simulink library "halout"  (R2021b)
settings: Solver=VariableStepAuto  StartTime=0.0  StopTime=10.0  RelTol=1e-3
undefined symbols (not defined in the file): C_TASK_5MS_S, FALSE, KHAL_CAN1FD1APS3E2E_flg, KHAL_CAN1FD1APS3TxReq_flg, KHAL_CAN1FD1VCU2E2E_flg, KHAL_CAN1FD1VCU2TxReq_flg, KHAL_CAN1FD1VCU3E2E_flg, KHAL_CAN1FD1VCU3TxReq_flg, KHAL_CAN1TxReq_flg, KHAL_CAN1VMCFCM1E2E_flg, KHAL_CAN1VMCFCM1TxReq_flg, KHAL_CAN2TxReq_flg, KHAL_CAN3FD3VCU1toNIDECTxReq_flg, KHAL_CAN3FD3VCU1TxReq_flg, KHAL_CAN3FD3VCU2E2E_flg, KHAL_CAN3FD3VCU2toNIDECE2E_flg, KHAL_CAN3FD3VCU2toNIDECTxReq_flg, KHAL_CAN3FD3VCU2TxReq_flg, KHAL_CAN3TxReq_flg, KHAL_CAN4FD4CE1000E2E_flg, KHAL_CAN4FD4CE1000TxReq_flg, KHAL_CAN4TxReq_flg, KHAL_CAN5TxReq_flg, KHAL_CAN6FD6APS3E2E_flg, KHAL_CAN6FD6APS3TxReq_flg, KHAL_CAN6FD6VCU2E2E_flg, KHAL_CAN6FD6VCU2TxReq_flg, KHAL_CAN6TxReq_flg, ONE_INT, TRUE, ZERO_INT
libraries: FVT_lib x551, simulink x244
(part 7 of 26)

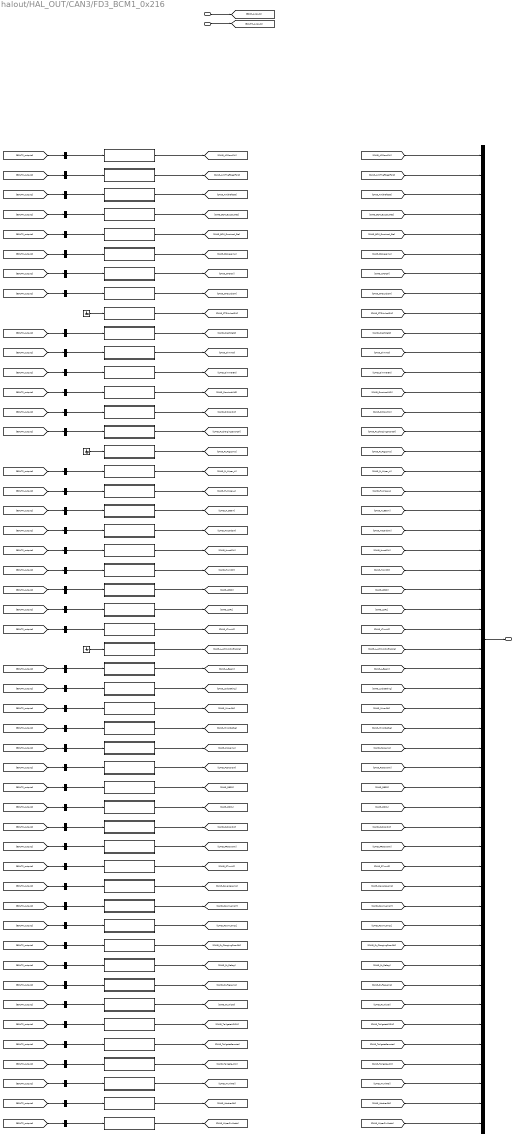
== system halout/HAL_OUT/CAN3/FD3_BCM1_0x216 ==
  BSCP_outputs : Inport  OutDataTypeStr=Bus: BSCP_outputs
  BOUTP_outputs : Inport  Port=2  OutDataTypeStr=Bus: BOUTP_outputs
  AllDoorSW : Subsystem
  AntiTheftSeatFold : Subsystem
  AntitheftSta : Subsystem
  BCMBuzzerReq : Subsystem
  BCMDoorLockSta : Subsystem
  BrakeLamp : Subsystem
  CTDCtrl : Subsystem
  CTDLockSW : Subsystem
  CTDUnlockSW : Subsystem
  CrashDetd : Subsystem
  Dimmer : Subsystem
  DimmerEN : Subsystem
  DoorLockIND : Subsystem
  DrDoorSW : Subsystem
  FrChargingDoorCtrl : Subsystem
  FrFogLamp : Subsystem
  FrWiperH : Subsystem
  FrWiperL : Subsystem
  Ground : Ground
  Ground1 : Ground
  Ground2 : Ground
  HBeam : Subsystem
  HazardSW : Subsystem
  HoodSW : Subsystem
  HornCtrl : Subsystem
  LAPMWdwEnable : Subsystem
  LBSD : Subsystem
  LBeam : Subsystem
  LDRL : Subsystem
  LTurnLP : Subsystem
  LockSetting : Subsystem
  MirrorCtrl : Subsystem
  MirrorDefog : Subsystem
  PosLamp : Subsystem
  PsDoorSW : Subsystem
  RBSD : Subsystem
  RDRL : Subsystem
  RLDoorSW : Subsystem
  RRDoorSW : Subsystem
  RTurnLP : Subsystem
  ReverseLamp : Subsystem
  RoomLampH : Subsystem
  RoomLampL : Subsystem
  RrChargingDoorCtrl : Subsystem
  RrDefog : Subsystem
  RrFogLamp : Subsystem
  RrWiper : Subsystem
  TailgateHDSW : Subsystem
  TailgateRemote : Subsystem
  TailgateSW : Subsystem
  TrunkRel : Subsystem
  WasherCtrl : Subsystem
  WiperFixMode : Subsystem
  bus_creator : BusCreator  Inputs=50  OutDataTypeStr=Bus: DT_CAN3_SG_FD3_BCM1  NonVirtualBus=on
  bus_selector : BusSelector  OutputSignals=VOUTP_AllDoorSW_flg
  bus_selector1 : BusSelector  OutputSignals=VOUTP_AntitheftSeatFlod_flg
  bus_selector10 : BusSelector  OutputSignals=VOUTP_DimmerEN_flg
  bus_selector11 : BusSelector  OutputSignals=VOUTP_DoorLockIND_flg
  bus_selector12 : BusSelector  OutputSignals=VOUTP_DrDoorSW_flg
  bus_selector13 : BusSelector  OutputSignals=VOUTP_FrChargingDoorCtrl_enum
  bus_selector14 : BusSelector  OutputSignals=VOUTP_FrWiperH_flg
  bus_selector15 : BusSelector  OutputSignals=VOUTP_FrWiperL_flg
  bus_selector16 : BusSelector  OutputSignals=VOUTP_HBeam_flg
  bus_selector17 : BusSelector  OutputSignals=VOUTP_HazardSW_flg
  bus_selector18 : BusSelector  OutputSignals=VOUTP_HoodSW_flg
  bus_selector19 : BusSelector  OutputSignals=VOUTP_HornCtrl_flg
  bus_selector2 : BusSelector  OutputSignals=VOUTP_AntitheftSta_enum
  bus_selector20 : BusSelector  OutputSignals=VOUTP_LBSD_flg
  bus_selector21 : BusSelector  OutputSignals=VOUTP_LDRL_flg
  bus_selector22 : BusSelector  OutputSignals=VOUTP_LTurnLP_flg
  bus_selector23 : BusSelector  OutputSignals=VOUTP_LBeam_flg
  bus_selector24 : BusSelector  OutputSignals=VOUTP_LockSetting_flg
  bus_selector25 : BusSelector  OutputSignals=VOUTP_MirrorCtrl_enum
  bus_selector26 : BusSelector  OutputSignals=VOUTP_MirrorDefog_flg
  bus_selector27 : BusSelector  OutputSignals=VOUTP_PosLamp_flg
  bus_selector28 : BusSelector  OutputSignals=VOUTP_PsDoorSW_flg
  bus_selector29 : BusSelector  OutputSignals=VOUTP_RBSD_flg
  bus_selector3 : BusSelector  OutputSignals=VOUTP_BCMBuzzerReq_flg
  bus_selector30 : BusSelector  OutputSignals=VOUTP_RDRL_flg
  bus_selector31 : BusSelector  OutputSignals=VOUTP_RLDoorSW_flg
  bus_selector32 : BusSelector  OutputSignals=VOUTP_RRDoorSW_flg
  bus_selector33 : BusSelector  OutputSignals=VOUTP_RTurnLP_flg
  bus_selector34 : BusSelector  OutputSignals=VOUTP_ReverseLamp_flg
  bus_selector35 : BusSelector  OutputSignals=VOUTP_RoomLampH_flg
  bus_selector36 : BusSelector  OutputSignals=VOUTP_RoomLampL_flg
  bus_selector37 : BusSelector  OutputSignals=VOUTP_RrChargingDoorCtrl_enum
  bus_selector38 : BusSelector  OutputSignals=VOUTP_RrDefog_flg
  bus_selector39 : BusSelector  OutputSignals=VOUTP_RrFogLamp_flg
  bus_selector4 : BusSelector  OutputSignals=VOUTP_BCMDoorLockSta_flg
  bus_selector40 : BusSelector  OutputSignals=VOUTP_RrWiper_flg
  bus_selector41 : BusSelector  OutputSignals=VOUTP_TailgateHDSW_flg
  bus_selector42 : BusSelector  OutputSignals=VOUTP_TailgateRemote_enum
  bus_selector43 : BusSelector  OutputSignals=VOUTP_TailgateSW_flg
  bus_selector44 : BusSelector  OutputSignals=VOUTP_TrunkRel_flg
  bus_selector45 : BusSelector  OutputSignals=VOUTP_WasherCtrl_enum
  bus_selector46 : BusSelector  OutputSignals=VOUTP_WiperFixMode_flg
  bus_selector5 : BusSelector  OutputSignals=VOUTP_BrakeLamp_flg
  bus_selector6 : BusSelector  OutputSignals=VOUTP_CTDCtrl_enum
  bus_selector7 : BusSelector  OutputSignals=VOUTP_CTDLockSW_flg
  bus_selector8 : BusSelector  OutputSignals=VOUTP_CrashDetd_flg
  bus_selector9 : BusSelector  OutputSignals=VOUTP_Dimmer_pct
  FD3_BCM1 : Outport
  wires:
  BSCP_outputs/1 -> [BSCP_outputs]
  BOUTP_outputs/1 -> [BOUTP_outputs]
  [CAN3_AllDoorSW] -> bus_creator/1  "CAN3_AllDoorSW"
  [CAN3_AntiTheftSeatFold] -> bus_creator/2  "CAN3_AntiTheftSeatFold"
  [CAN3_AntitheftSta] -> bus_creator/3  "CAN3_AntitheftSta"
  [CAN3_BCM_Buzzer_Req] -> bus_creator/4  "CAN3_BCM_Buzzer_Req"
  [CAN3_BCM_DoorLock_Sta] -> bus_creator/5  "CAN3_BCM_DoorLock_Sta"
  [CAN3_BrakeLamp] -> bus_creator/6  "CAN3_BrakeLamp"
  [CAN3_CTDCtrl] -> bus_creator/7  "CAN3_CTDCtrl"
  [CAN3_CTDLockSW] -> bus_creator/8  "CAN3_CTDLockSW"
  [CAN3_CTDUnlockSW] -> bus_creator/9  "CAN3_CTDUnlockSW"
  [CAN3_CrashDetd] -> bus_creator/10  "CAN3_CrashDetd"
  [CAN3_Dimmer] -> bus_creator/11  "CAN3_Dimmer"
  [CAN3_DimmerEN] -> bus_creator/12  "CAN3_DimmerEN"
  [CAN3_DoorLockIND] -> bus_creator/13  "CAN3_DoorLockIND"
  [CAN3_DrDoorSW] -> bus_creator/14  "CAN3_DrDoorSW"
  [CAN3_Fr_ChargingDoorCtrl] -> bus_creator/15  "CAN3_Fr_ChargingDoorCtrl"
  [CAN3_Fr_FogLamp] -> bus_creator/16  "CAN3_Fr_FogLamp"
  [CAN3_Fr_Wiper_H] -> bus_creator/17  "CAN3_Fr_Wiper_H"
  [CAN3_Fr_Wiper_L] -> bus_creator/18  "CAN3_Fr_Wiper_L"
  [CAN3_H_Beam] -> bus_creator/19  "CAN3_H_Beam"
  [CAN3_HazardSW] -> bus_creator/20  "CAN3_HazardSW"
  [CAN3_HoodSW] -> bus_creator/21  "CAN3_HoodSW"
  [CAN3_HornCtrl] -> bus_creator/22  "CAN3_HornCtrl"
  [CAN3_LBSD] -> bus_creator/23  "CAN3_LBSD"
  [CAN3_LDRL] -> bus_creator/24  "CAN3_LDRL"
  [CAN3_LTurnLP] -> bus_creator/25  "CAN3_LTurnLP"
  [CAN3_L_APM_WdwEnable] -> bus_creator/26  "CAN3_L_APM_WdwEnable"
  [CAN3_L_Beam] -> bus_creator/27  "CAN3_L_Beam"
  [CAN3_LockSetting] -> bus_creator/28  "CAN3_LockSetting"
  [CAN3_MirrorCtrl] -> bus_creator/29  "CAN3_MirrorCtrl"
  [CAN3_MirrorDefog] -> bus_creator/30  "CAN3_MirrorDefog"
  [CAN3_PosLamp] -> bus_creator/31  "CAN3_PosLamp"
  [CAN3_PsDoorSW] -> bus_creator/32  "CAN3_PsDoorSW"
  [CAN3_RBSD] -> bus_creator/33  "CAN3_RBSD"
  [CAN3_RDRL] -> bus_creator/34  "CAN3_RDRL"
  [CAN3_RLDoorSW] -> bus_creator/35  "CAN3_RLDoorSW"
  [CAN3_RRDoorSW] -> bus_creator/36  "CAN3_RRDoorSW"
  [CAN3_RTurnLP] -> bus_creator/37  "CAN3_RTurnLP"
  [CAN3_ReverseLamp] -> bus_creator/38  "CAN3_ReverseLamp"
  [CAN3_RoomLampH] -> bus_creator/39  "CAN3_RoomLampH"
  [CAN3_RoomLampL] -> bus_creator/40  "CAN3_RoomLampL"
  [CAN3_Rr_ChargingDoorCtrl] -> bus_creator/41  "CAN3_Rr_ChargingDoorCtrl"
  [CAN3_Rr_Defog] -> bus_creator/42  "CAN3_Rr_Defog"
  [CAN3_Rr_FogLamp] -> bus_creator/43  "CAN3_Rr_FogLamp"
  [CAN3_Rr_Wiper] -> bus_creator/44  "CAN3_Rr_Wiper"
  [CAN3_TailgateHDSW] -> bus_creator/45  "CAN3_TailgateHDSW"
  [CAN3_TailgateRemote] -> bus_creator/46  "CAN3_TailgateRemote"
  [CAN3_Tailgate_SW] -> bus_creator/47  "CAN3_Tailgate_SW"
  [CAN3_TrunkRel] -> bus_creator/48  "CAN3_TrunkRel"
  [CAN3_WasherCtrl] -> bus_creator/49  "CAN3_WasherCtrl"
  [CAN3_WiperFixMode] -> bus_creator/50  "CAN3_WiperFixMode"
  bus_creator/1 -> FD3_BCM1/1
  AllDoorSW/1(CAN3_AllDoorSW) -> [CAN3_AllDoorSW]
  AntiTheftSeatFold/1(CAN3_AntiTheftSeatFold) -> [CAN3_AntiTheftSeatFold]
  AntitheftSta/1(CAN3_AntitheftSta) -> [CAN3_AntitheftSta]
  BCMBuzzerReq/1(CAN3_BCM_Buzzer_Req) -> [CAN3_BCM_Buzzer_Req]
  BCMDoorLockSta/1(CAN3_BCM_DoorLock_Sta) -> [CAN3_BCM_DoorLock_Sta]
  BrakeLamp/1(CAN3_BrakeLamp) -> [CAN3_BrakeLamp]
  CTDCtrl/1(CAN3_CTDCtrl) -> [CAN3_CTDCtrl]
  CTDLockSW/1(CAN3_CTDLockSW) -> [CAN3_CTDLockSW]
  CTDUnlockSW/1(CAN3_CTDUnlockSW) -> [CAN3_CTDUnlockSW]
  CrashDetd/1(CAN3_CrashDetd) -> [CAN3_CrashDetd]
  Dimmer/1(CAN3_Dimmer) -> [CAN3_Dimmer]
  DimmerEN/1(CAN3_DimmerEN) -> [CAN3_DimmerEN]
  DoorLockIND/1(CAN3_DoorLockIND) -> [CAN3_DoorLockIND]
  DrDoorSW/1(CAN3_DrDoorSW) -> [CAN3_DrDoorSW]
  FrChargingDoorCtrl/1(CAN3_Fr_ChargingDoorCtrl) -> [CAN3_Fr_ChargingDoorCtrl]
  FrFogLamp/1(CAN3_Fr_FogLamp) -> [CAN3_Fr_FogLamp]
  FrWiperH/1(CAN3_Fr_Wiper_H) -> [CAN3_Fr_Wiper_H]
  FrWiperL/1(CAN3_Fr_Wiper_L) -> [CAN3_Fr_Wiper_L]
  HBeam/1(CAN3_H_Beam) -> [CAN3_H_Beam]
  HazardSW/1(CAN3_HazardSW) -> [CAN3_HazardSW]
  HoodSW/1(CAN3_HoodSW) -> [CAN3_HoodSW]
  HornCtrl/1(CAN3_HornCtrl) -> [CAN3_HornCtrl]
  LBSD/1(CAN3_LBSD) -> [CAN3_LBSD]
  LDRL/1(CAN3_LDRL) -> [CAN3_LDRL]
  LTurnLP/1(CAN3_LTurnLP) -> [CAN3_LTurnLP]
  LAPMWdwEnable/1(CAN3_L_APM_WdwEnable) -> [CAN3_L_APM_WdwEnable]
  LBeam/1(CAN3_L_Beam) -> [CAN3_L_Beam]
  LockSetting/1(CAN3_LockSetting) -> [CAN3_LockSetting]
  MirrorCtrl/1(CAN3_MirrorCtrl) -> [CAN3_MirrorCtrl]
  MirrorDefog/1(CAN3_MirrorDefog) -> [CAN3_MirrorDefog]
  PosLamp/1(CAN3_PosLamp) -> [CAN3_PosLamp]
  PsDoorSW/1(CAN3_PsDoorSW) -> [CAN3_PsDoorSW]
  RBSD/1(CAN3_RBSD) -> [CAN3_RBSD]
  RDRL/1(CAN3_RDRL) -> [CAN3_RDRL]
  RLDoorSW/1(CAN3_RLDoorSW) -> [CAN3_RLDoorSW]
  RRDoorSW/1(CAN3_RRDoorSW) -> [CAN3_RRDoorSW]
  RTurnLP/1(CAN3_RTurnLP) -> [CAN3_RTurnLP]
  ReverseLamp/1(CAN3_ReverseLamp) -> [CAN3_ReverseLamp]
  RoomLampH/1(CAN3_RoomLampH) -> [CAN3_RoomLampH]
  RoomLampL/1(CAN3_RoomLampL) -> [CAN3_RoomLampL]
  RrChargingDoorCtrl/1(CAN3_Rr_ChargingDoorCtrl) -> [CAN3_Rr_ChargingDoorCtrl]
  RrDefog/1(CAN3_Rr_Defog) -> [CAN3_Rr_Defog]
  RrFogLamp/1(CAN3_Rr_FogLamp) -> [CAN3_Rr_FogLamp]
  RrWiper/1(CAN3_Rr_Wiper) -> [CAN3_Rr_Wiper]
  TailgateHDSW/1(CAN3_TailgateHDSW) -> [CAN3_TailgateHDSW]
  TailgateRemote/1(CAN3_TailgateRemote) -> [CAN3_TailgateRemote]
  TailgateSW/1(CAN3_Tailgate_SW) -> [CAN3_Tailgate_SW]
  TrunkRel/1(CAN3_TrunkRel) -> [CAN3_TrunkRel]
  WasherCtrl/1(CAN3_WasherCtrl) -> [CAN3_WasherCtrl]
  WiperFixMode/1(CAN3_WiperFixMode) -> [CAN3_WiperFixMode]
  bus_selector/1 -> AllDoorSW/1(AllDoorSW)  "<VOUTP_AllDoorSW_flg>"
  [BOUTP_outputs] -> bus_selector/1
  bus_selector1/1 -> AntiTheftSeatFold/1(AntiTheftSeatFold)  "<VOUTP_AntitheftSeatFlod_flg>"
  [BOUTP_outputs] -> bus_selector1/1
  bus_selector2/1 -> AntitheftSta/1(AntitheftSta)  "<VOUTP_AntitheftSta_enum>"
  [BOUTP_outputs] -> bus_selector2/1
  bus_selector3/1 -> BCMBuzzerReq/1(BCMBuzzerReq)  "<VOUTP_BCMBuzzerReq_flg>"
  [BOUTP_outputs] -> bus_selector3/1
  bus_selector4/1 -> BCMDoorLockSta/1(BCMDoorLockSta)  "<VOUTP_BCMDoorLockSta_flg>"
  [BOUTP_outputs] -> bus_selector4/1
  bus_selector5/1 -> BrakeLamp/1(BrakeLamp)  "<VOUTP_BrakeLamp_flg>"
  [BOUTP_outputs] -> bus_selector5/1
  bus_selector6/1 -> CTDCtrl/1(CTDCtrl)  "<VOUTP_CTDCtrl_enum>"
  [BOUTP_outputs] -> bus_selector6/1
  bus_selector7/1 -> CTDLockSW/1(CTDLockSW)  "<VOUTP_CTDLockSW_flg>"
  [BOUTP_outputs] -> bus_selector7/1
  Ground/1 -> CTDUnlockSW/1(CTDUnlockSW)
  bus_selector8/1 -> CrashDetd/1(CrashDetd)  "<VOUTP_CrashDetd_flg>"
  [BOUTP_outputs] -> bus_selector8/1
  bus_selector9/1 -> Dimmer/1(Dimmer)  "<VOUTP_Dimmer_pct>"
  [BOUTP_outputs] -> bus_selector9/1
  bus_selector10/1 -> DimmerEN/1(DimmerEN)  "<VOUTP_DimmerEN_flg>"
  [BOUTP_outputs] -> bus_selector10/1
  bus_selector11/1 -> DoorLockIND/1(DoorLockIND)  "<VOUTP_DoorLockIND_flg>"
  [BOUTP_outputs] -> bus_selector11/1
  bus_selector12/1 -> DrDoorSW/1(DrDoorSW)  "<VOUTP_DrDoorSW_flg>"
  [BOUTP_outputs] -> bus_selector12/1
  bus_selector13/1 -> FrChargingDoorCtrl/1(FrChargingDoorCtrl)  "<VOUTP_FrChargingDoorCtrl_enum>"
  [BOUTP_outputs] -> bus_selector13/1
  Ground1/1 -> FrFogLamp/1(FrFogLamp)
  bus_selector14/1 -> FrWiperH/1(FrWiperH)  "<VOUTP_FrWiperH_flg>"
  [BOUTP_outputs] -> bus_selector14/1
  bus_selector15/1 -> FrWiperL/1(FrWiperL)  "<VOUTP_FrWiperL_flg>"
  [BOUTP_outputs] -> bus_selector15/1
  bus_selector16/1 -> HBeam/1(HBeam)  "<VOUTP_HBeam_flg>"
  [BOUTP_outputs] -> bus_selector16/1
  bus_selector17/1 -> HazardSW/1(HazardSW)  "<VOUTP_HazardSW_flg>"
  [BOUTP_outputs] -> bus_selector17/1
  bus_selector18/1 -> HoodSW/1(HoodSW)  "<VOUTP_HoodSW_flg>"
  [BOUTP_outputs] -> bus_selector18/1
  bus_selector19/1 -> HornCtrl/1(HornCtrl)  "<VOUTP_HornCtrl_flg>"
  [BOUTP_outputs] -> bus_selector19/1
  bus_selector20/1 -> LBSD/1(LBSD)  "<VOUTP_LBSD_flg>"
  [BOUTP_outputs] -> bus_selector20/1
  bus_selector21/1 -> LDRL/1(LDRL)  "<VOUTP_LDRL_flg>"
  [BOUTP_outputs] -> bus_selector21/1
  bus_selector22/1 -> LTurnLP/1(LTurnLP)  "<VOUTP_LTurnLP_flg>"
  [BOUTP_outputs] -> bus_selector22/1
  Ground2/1 -> LAPMWdwEnable/1(LAPMWdwEnable)
  bus_selector23/1 -> LBeam/1(LBeam)  "<VOUTP_LBeam_flg>"
  [BOUTP_outputs] -> bus_selector23/1
  bus_selector24/1 -> LockSetting/1(LockSetting)  "<VOUTP_LockSetting_flg>"
  [BOUTP_outputs] -> bus_selector24/1
  bus_selector25/1 -> MirrorCtrl/1(MirrorCtrl)  "<VOUTP_MirrorCtrl_enum>"
  [BOUTP_outputs] -> bus_selector25/1
  bus_selector26/1 -> MirrorDefog/1(MirrorDefog)  "<VOUTP_MirrorDefog_flg>"
  [BOUTP_outputs] -> bus_selector26/1
  bus_selector27/1 -> PosLamp/1(PosLamp)  "<VOUTP_PosLamp_flg>"
  [BOUTP_outputs] -> bus_selector27/1
  bus_selector28/1 -> PsDoorSW/1(PsDoorSW)  "<VOUTP_PsDoorSW_flg>"
  [BOUTP_outputs] -> bus_selector28/1
  bus_selector29/1 -> RBSD/1(RBSD)  "<VOUTP_RBSD_flg>"
  [BOUTP_outputs] -> bus_selector29/1
  bus_selector30/1 -> RDRL/1(RDRL)  "<VOUTP_RDRL_flg>"
  [BOUTP_outputs] -> bus_selector30/1
  bus_selector31/1 -> RLDoorSW/1(RLDoorSW)  "<VOUTP_RLDoorSW_flg>"
  [BOUTP_outputs] -> bus_selector31/1
  bus_selector32/1 -> RRDoorSW/1(RRDoorSW)  "<VOUTP_RRDoorSW_flg>"
  [BOUTP_outputs] -> bus_selector32/1
  bus_selector33/1 -> RTurnLP/1(RTurnLP)  "<VOUTP_RTurnLP_flg>"
  [BOUTP_outputs] -> bus_selector33/1
  bus_selector34/1 -> ReverseLamp/1(ReverseLamp)  "<VOUTP_ReverseLamp_flg>"
  [BOUTP_outputs] -> bus_selector34/1
  bus_selector35/1 -> RoomLampH/1(RoomLampH)  "<VOUTP_RoomLampH_flg>"
  [BOUTP_outputs] -> bus_selector35/1
  bus_selector36/1 -> RoomLampL/1(RoomLampL)  "<VOUTP_RoomLampL_flg>"
  [BOUTP_outputs] -> bus_selector36/1
  bus_selector37/1 -> RrChargingDoorCtrl/1(RrChargingDoorCtrl)  "<VOUTP_RrChargingDoorCtrl_enum>"
  [BOUTP_outputs] -> bus_selector37/1
  bus_selector38/1 -> RrDefog/1(RrDefog)  "<VOUTP_RrDefog_flg>"
  [BOUTP_outputs] -> bus_selector38/1
  bus_selector39/1 -> RrFogLamp/1(RrFogLamp)  "<VOUTP_RrFogLamp_flg>"
  [BOUTP_outputs] -> bus_selector39/1
  bus_selector40/1 -> RrWiper/1(RrWiper)  "<VOUTP_RrWiper_flg>"
  [BOUTP_outputs] -> bus_selector40/1
  bus_selector41/1 -> TailgateHDSW/1(TailgateHDSW)  "<VOUTP_TailgateHDSW_flg>"
  [BOUTP_outputs] -> bus_selector41/1
  bus_selector42/1 -> TailgateRemote/1(TailgateRemote)  "<VOUTP_TailgateRemote_enum>"
  [BOUTP_outputs] -> bus_selector42/1
  bus_selector43/1 -> TailgateSW/1(TailgateSW)  "<VOUTP_TailgateSW_flg>"
  [BOUTP_outputs] -> bus_selector43/1
  bus_selector44/1 -> TrunkRel/1(TrunkRel)  "<VOUTP_TrunkRel_flg>"
  [BOUTP_outputs] -> bus_selector44/1
  bus_selector45/1 -> WasherCtrl/1(WasherCtrl)  "<VOUTP_WasherCtrl_enum>"
  [BOUTP_outputs] -> bus_selector45/1
  bus_selector46/1 -> WiperFixMode/1(WiperFixMode)  "<VOUTP_WiperFixMode_flg>"
  [BOUTP_outputs] -> bus_selector46/1

== system halout/HAL_OUT/CAN3/FD3_C100_0_0x182 ==
  BSCP_outputs : Inport  OutDataTypeStr=Bus: BSCP_outputs
  BOUTP_outputs : Inport  Port=2  OutDataTypeStr=Bus: BOUTP_outputs
  BatteryMode : Subsystem
  FrCoolantflow : Subsystem
  FrCoolanttemp : Subsystem
  Ground{,1..4} (5 alike) : Ground
  RrCoolantflow : Subsystem
  RrCoolanttemp : Subsystem
  bus_creator : BusCreator  Inputs=6  OutDataTypeStr=Bus: DT_CAN3_SG_FD3_C100_0  NonVirtualBus=on
  bus_selector : BusSelector  OutputSignals=VOUTP_BatteryMode_enum
  sigCbnPTCPwrAct : Subsystem
  FD3_C100_0 : Outport
  wires:
  BSCP_outputs/1 -> [BSCP_outputs]
  BOUTP_outputs/1 -> [BOUTP_outputs]
  [CAN3_BatteryMode] -> bus_creator/1  "CAN3_BatteryMode"
  [CAN3_Fr_Coolantflow] -> bus_creator/2  "CAN3_Fr_Coolantflow"
  [CAN3_Fr_Coolanttemp] -> bus_creator/3  "CAN3_Fr_Coolanttemp"
  [CAN3_Rr_Coolantflow] -> bus_creator/4  "CAN3_Rr_Coolantflow"
  [CAN3_Rr_Coolanttemp] -> bus_creator/5  "CAN3_Rr_Coolanttemp"
  [CAN3_sigCbnPTCPwrAct] -> bus_creator/6  "CAN3_sigCbnPTCPwrAct"
  bus_creator/1 -> FD3_C100_0/1
  BatteryMode/1(CAN3_BatteryMode) -> [CAN3_BatteryMode]
  FrCoolantflow/1(CAN3_Fr_Coolantflow) -> [CAN3_Fr_Coolantflow]
  FrCoolanttemp/1(CAN3_Fr_Coolanttemp) -> [CAN3_Fr_Coolanttemp]
  RrCoolantflow/1(CAN3_Rr_Coolantflow) -> [CAN3_Rr_Coolantflow]
  RrCoolanttemp/1(CAN3_Rr_Coolanttemp) -> [CAN3_Rr_Coolanttemp]
  sigCbnPTCPwrAct/1(CAN3_sigCbnPTCPwrAct) -> [CAN3_sigCbnPTCPwrAct]
  bus_selector/1 -> BatteryMode/1(BatteryMode)  "<VOUTP_BatteryMode_enum>"
  [BOUTP_outputs] -> bus_selector/1
  Ground/1 -> FrCoolantflow/1(FrCoolantflow)
  Ground1/1 -> FrCoolanttemp/1(FrCoolanttemp)
  Ground2/1 -> RrCoolantflow/1(RrCoolantflow)
  Ground3/1 -> RrCoolanttemp/1(RrCoolanttemp)
  Ground4/1 -> sigCbnPTCPwrAct/1(sigCbnPTCPwrAct)

== system halout/HAL_OUT/CAN3/FD3_V2L1_0x374 ==
  BSCP_outputs : Inport  OutDataTypeStr=Bus: BSCP_outputs
  BOUTP_outputs : Inport  Port=2  OutDataTypeStr=Bus: BOUTP_outputs
  FDCV2LOBCExtrV2LCmd : Subsystem
  FDCV2LOBCIntrV2LCmd : Subsystem
  Ground : Ground
  ReqOBCV2LEna : Subsystem
  ReqV2LIVIPopup : Subsystem
  ReqV2LSwOn : Subsystem
  bus_creator : BusCreator  Inputs=5  OutDataTypeStr=Bus: DT_CAN3_SG_FD3_V2L1  NonVirtualBus=on
  bus_selector : BusSelector  OutputSignals=VOUTP_ReqOBCExtrV2LEna_enum
  bus_selector1 : BusSelector  OutputSignals=VOUTP_ReqOBCIntrV2LEna_enum
  bus_selector2 : BusSelector  OutputSignals=VOUTP_ReqOBCV2LEna_enum
  bus_selector3 : BusSelector  OutputSignals=VOUTP_ReqV2LIVIPopup_enum
  FD3_V2L1 : Outport
  wires:
  BSCP_outputs/1 -> [BSCP_outputs]
  BOUTP_outputs/1 -> [BOUTP_outputs]
  [CAN3_FDC_V2L_OBCExtrV2L_Cmd] -> bus_creator/1  "CAN3_FDC_V2L_OBCExtrV2L_Cmd"
  [CAN3_FDC_V2L_OBCIntrV2L_Cmd] -> bus_creator/2  "CAN3_FDC_V2L_OBCIntrV2L_Cmd"
  [CAN3_Req_OBCV2LEna] -> bus_creator/3  "CAN3_Req_OBCV2LEna"
  [CAN3_Req_V2LSwOn] -> bus_creator/4  "CAN3_Req_V2LSwOn"
  [CAN3_Req_V2L_IVI_Popup] -> bus_creator/5  "CAN3_Req_V2L_IVI_Popup"
  bus_creator/1 -> FD3_V2L1/1
  FDCV2LOBCExtrV2LCmd/1(CAN3_FDC_V2L_OBCExtrV2L_Cmd) -> [CAN3_FDC_V2L_OBCExtrV2L_Cmd]
  FDCV2LOBCIntrV2LCmd/1(CAN3_FDC_V2L_OBCIntrV2L_Cmd) -> [CAN3_FDC_V2L_OBCIntrV2L_Cmd]
  ReqOBCV2LEna/1(CAN3_Req_OBCV2LEna) -> [CAN3_Req_OBCV2LEna]
  ReqV2LSwOn/1(CAN3_Req_V2LSwOn) -> [CAN3_Req_V2LSwOn]
  ReqV2LIVIPopup/1(CAN3_Req_V2L_IVI_Popup) -> [CAN3_Req_V2L_IVI_Popup]
  bus_selector/1 -> FDCV2LOBCExtrV2LCmd/1(FDCV2LOBCExtrV2LCmd)  "<VOUTP_ReqOBCExtrV2LEna_enum>"
  [BOUTP_outputs] -> bus_selector/1
  bus_selector1/1 -> FDCV2LOBCIntrV2LCmd/1(FDCV2LOBCIntrV2LCmd)  "<VOUTP_ReqOBCIntrV2LEna_enum>"
  [BOUTP_outputs] -> bus_selector1/1
  bus_selector2/1 -> ReqOBCV2LEna/1(ReqOBCV2LEna)  "<VOUTP_ReqOBCV2LEna_enum>"
  [BOUTP_outputs] -> bus_selector2/1
  Ground/1 -> ReqV2LSwOn/1(ReqV2LSwOn)
  bus_selector3/1 -> ReqV2LIVIPopup/1(ReqV2LIVIPopup)  "<VOUTP_ReqV2LIVIPopup_enum>"
  [BOUTP_outputs] -> bus_selector3/1

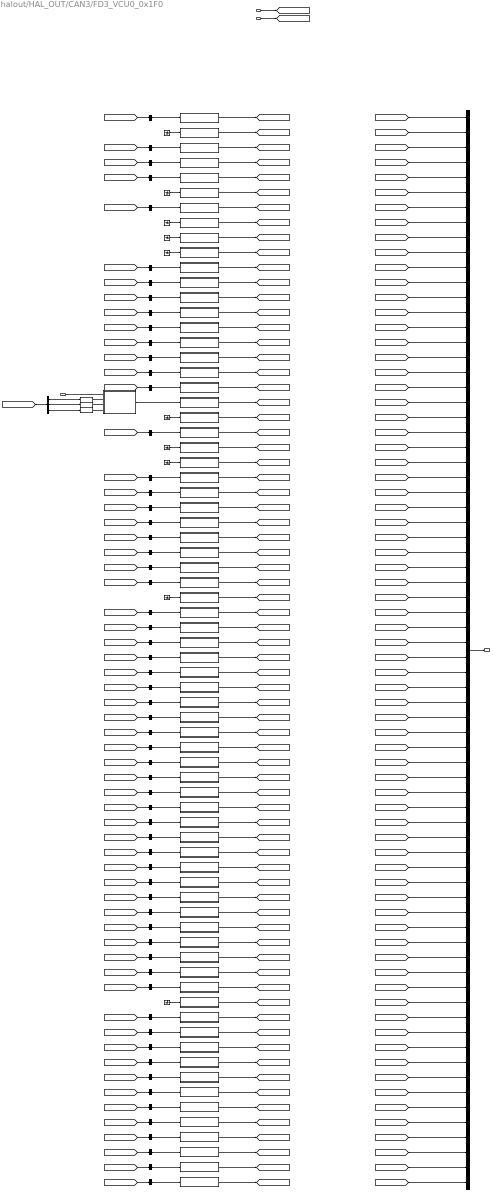
== system halout/HAL_OUT/CAN3/FD3_VCU0_0x1F0 ==
  BSCP_outputs : Inport  OutDataTypeStr=Bus: BSCP_outputs
  BOUTP_outputs : Inport  Port=2  OutDataTypeStr=Bus: BOUTP_outputs
  s8_AcoreReadyToSleep : Inport  Port=3
  Data Type Conversion : DataTypeConversion  OutDataTypeStr=uint8
  Data Type Conversion1 : DataTypeConversion  OutDataTypeStr=uint8
  Data Type Conversion2 : DataTypeConversion  OutDataTypeStr=uint8
  EVCCAplusPwrUpReq : Subsystem
  FDADC12VDet : Subsystem
  FDADC12VDetAvg : Subsystem
  FDCSYSPmicBootPath : Subsystem
  FDCVCUActMaxSlideRateSta : Subsystem
  FDCVCUAllowMovThdOTASta : Subsystem
  FDCVCUBOSEnableSta : Subsystem
  FDCVCUBrakeSigMatrixSta : Subsystem
  FDCVCUBrkPedalPosStaSta : Subsystem
  FDCVCUCANBrkSW2StaSta : Subsystem
  FDCVCUDTCCarouselSta : Subsystem
  FDCVCUEAPS1MinSta : Subsystem
  FDCVCUEAPS1RawSta : Subsystem
  FDCVCUEAPS2MinSta : Subsystem
  FDCVCUEAPS2RawSta : Subsystem
  FDCVCUForcePCmd : Subsystem
  FDCVCUFrFirstOrderInpTs : Subsystem
  FDCVCUFrRateLimitDecSta : Subsystem
  FDCVCUFrRateLimitIncSta : Subsystem
  FDCVCULVChrgFreqCntSta : Subsystem
  FDCVCULVStaDropQukCntSta : Subsystem
  FDCVCULowIdleAccPedalSta : Subsystem
  FDCVCUOTAPwrReqOFFChkSta : Subsystem
  FDCVCUOTAPwrReqStdChkSta : Subsystem
  FDCVCUPwrReqOTASta : Subsystem
  FDCVCURWDRDCActiveSta : Subsystem
  FDCVCURegenTqLimitEnSta : Subsystem
  FDCVCURrFirstOrderInpTs : Subsystem
  FDCVCURrRateLimitDecSta : Subsystem
  FDCVCURrRateLimitIncSta : Subsystem
  FDCVCUSlideRegenLimTqSta : Subsystem
  FDCVCUVehActSpdSta : Subsystem
  FDCVCUVehMalfunLevelSta : Subsystem
  FDCVMCActStESCYawSta : Subsystem
  FDCVMCLongAccSta : Subsystem
  FrTqSource : Subsystem
  Ground{,1..4,8..12} (10 alike) : Ground
  HVRlyOpFail : Subsystem
  HVTHCMSysAvail : Subsystem
  LVBattChrgtimeAct : Subsystem
  LVBattVoltSta : Subsystem
  LVChrgHoldTAct : Subsystem
  LVSilentChrgLv : Subsystem
  LVSilentChrgReq : Subsystem
  LVSilentChrgSta : Subsystem
  MCUActDisFail : Subsystem
  PMMAllowECUSleep : Subsystem
  PmicBootReason : Subsystem
  PowerDownFault : Subsystem
  PowerDownState : Subsystem
  PowerUpFault : Subsystem
  PowerUpState : Subsystem
  PwrDownReq : Subsystem
  PwrStaConstraint : Subsystem
  PwrStaONTOIVIPopReq : Subsystem
  PwrStaONTOIVIPopT : Subsystem
  PwrStaSelect : Subsystem
  PwrStaTOSta : Subsystem
  PwrUpReq : Subsystem
  RrTqSource : Subsystem
  SchedChgTOSta : Subsystem
  SilentChkAllowSleep : Subsystem
  Subsystem : Subsystem
  SysAllowReadySta : Subsystem
  SysPwrSta : Subsystem
  TCountSta : Subsystem
  TimerAllowSleep : Subsystem
  VCUBrkSWSta : Subsystem
  VCUFLDoorSta : Subsystem
  VCUFRDoorSta : Subsystem
  VCURLDoorSta : Subsystem
  VCURRDoorSta : Subsystem
  VehHVPwrAvail4THCM : Subsystem
  WisrBootReason : Subsystem
  bus_creator : BusCreator  Inputs=72  OutDataTypeStr=Bus: DT_CAN3_SG_FD3_VCU0  NonVirtualBus=on
  bus_selector : BusSelector  OutputSignals=VOUTP_EvccAplusPwrUpReq_flg
  bus_selector1 : BusSelector  OutputSignals=VOUTP_FDADC12VDetAvg_mV
  bus_selector10 : BusSelector  OutputSignals=VOUTP_FrRateLimitDec_Nm
  bus_selector11 : BusSelector  OutputSignals=VOUTP_FrRateLimitInc_Nm
  bus_selector12 : BusSelector  OutputSignals=VOUTP_LowIdleAccPedal_flg
  bus_selector13 : BusSelector  OutputSignals=VOUTP_PwrReq_OTA_enum
  bus_selector14 : BusSelector  OutputSignals=VOUTP_RDCActive_enum
  bus_selector15 : BusSelector  OutputSignals=VOUTP_RegenTqLimitEn_flg
  bus_selector16 : BusSelector  OutputSignals=VOUTP_RrFirstOrderInpTs_c
  bus_selector17 : BusSelector  OutputSignals=VOUTP_RrRateLimitDec_Nm
  bus_selector18 : BusSelector  OutputSignals=VOUTP_RrRateLimitInc_Nm
  bus_selector19 : BusSelector  OutputSignals=VOUTP_SlideRegenLimTq_Nm
  bus_selector2 : BusSelector  OutputSignals=VOUTP_PmicBootPath_raw32
  bus_selector20 : BusSelector  OutputSignals=VOUTP_VehActSpd_kph
  bus_selector21 : BusSelector  OutputSignals=VOUTP_ActStESCYaw_Dps
  bus_selector22 : BusSelector  OutputSignals=VOUTP_LongAcc_Gps
  bus_selector23 : BusSelector  OutputSignals=VOUTP_TqSourceFr_enum
  bus_selector24 : BusSelector  OutputSignals=VOUTP_HVRlyOpFail_flg
  bus_selector25 : BusSelector  OutputSignals=VOUTP_HVTHCMSysAvail_enum
  bus_selector26 : BusSelector  OutputSignals=VOUTP_LVBattChrgTimeCnt_s
  bus_selector27 : BusSelector  OutputSignals=VOUTP_LVBattVoltSta_enum
  bus_selector28 : BusSelector  OutputSignals=VOUTP_LVChrgHoldTtimer_s
  bus_selector29 : BusSelector  OutputSignals=VOUTP_LVSilentChrgLv_enum
  bus_selector3 : BusSelector  OutputSignals=VOUTP_MaxWhlSlideRate_pct
  bus_selector30 : BusSelector  OutputSignals=VOUTP_LVSilentChrgReq_flg
  bus_selector31 : BusSelector  OutputSignals=VOUTP_LVSilentChrgSta_enum
  bus_selector32 : BusSelector  OutputSignals=VOUTP_MCUActDisFail_flg
  bus_selector33 : BusSelector  OutputSignals=VOUTP_PMMAllowECUSleep_flg
  bus_selector34 : BusSelector  OutputSignals=VOUTP_PmicBootReason_enum
  bus_selector35 : BusSelector  OutputSignals=VOUTP_PowerDownFault_enum
  bus_selector36 : BusSelector  OutputSignals=VOUTP_PowerDownState_enum
  bus_selector37 : BusSelector  OutputSignals=VOUTP_PowerUpFault_enum
  bus_selector38 : BusSelector  OutputSignals=VOUTP_PowerUpState_enum
  bus_selector39 : BusSelector  OutputSignals=VOUTP_PwrDownReq_enum
  bus_selector4 : BusSelector  OutputSignals=VOUTP_BOSEnable_flg
  bus_selector40 : BusSelector  OutputSignals=VOUTP_PwrStaConstraint_enum
  bus_selector41 : BusSelector  OutputSignals=VOUTP_PwrStaONTOPopReq_flg
  bus_selector42 : BusSelector  OutputSignals=VOUTP_IVIPwrStaONTOPopT_s
  bus_selector43 : BusSelector  OutputSignals=VOUTP_PwrStaSelect_enum
  bus_selector44 : BusSelector  OutputSignals=VOUTP_PwrStaTOSta_enum
  bus_selector45 : BusSelector  OutputSignals=VOUTP_PwrUpReq_enum
  bus_selector46 : BusSelector  OutputSignals=VOUTP_TqSourceRr_enum
  bus_selector47 : BusSelector  OutputSignals=VOUTP_SilentChkAllowSleep_flg
  bus_selector48 : BusSelector  OutputSignals=VOUTP_SysAllowReadySta_flg
  bus_selector49 : BusSelector  OutputSignals=VOUTP_SysPowerMode_enum
  bus_selector5 : BusSelector  OutputSignals=VOUTP_DTCDetect_enum
  bus_selector50 : BusSelector  OutputSignals=VOUTP_TCountSta_enum
  bus_selector51 : BusSelector  OutputSignals=VOUTP_TimerAllowSleep_flg
  bus_selector52 : BusSelector  OutputSignals=VOUTP_VCUBrkSWSta_enum
  bus_selector53 : BusSelector  OutputSignals=VOUTP_VCUFLDoorSta_flg
  bus_selector54 : BusSelector  OutputSignals=VOUTP_VCUFRDoorSta_flg
  bus_selector55 : BusSelector  OutputSignals=VOUTP_VCURLDoorSta_flg
  bus_selector56 : BusSelector  OutputSignals=VOUTP_VCURRDoorSta_flg
  bus_selector57 : BusSelector  OutputSignals=VOUTP_VehHVPwrAvail4THCM_W
  bus_selector58 : BusSelector  OutputSignals=VOUTP_WisrBootReason_raw32
  bus_selector59 : BusSelector  OutputSignals=VOUTP_CurrentNmState_enum,VOUTP_OTAPwrReqOFFChkSta_enum,VOUTP_OTAPwrReqStdChkSta_enum
  bus_selector6 : BusSelector  OutputSignals=VOUTP_EAPS1MIN_pct
  bus_selector60 : BusSelector  OutputSignals=VOUTP_EAPS2RAW_pct
  bus_selector61 : BusSelector  OutputSignals=VOUTP_EAPS1RAW_pct
  bus_selector7 : BusSelector  OutputSignals=VOUTP_EAPS2MIN_pct
  bus_selector8 : BusSelector  OutputSignals=VOUTP_ForceP_flg
  bus_selector9 : BusSelector  OutputSignals=VOUTP_FrFirstOrderInpTs_c
  FD3_VCU0 : Outport
  wires:
  BSCP_outputs/1 -> [BSCP_outputs]
  BOUTP_outputs/1 -> [BOUTP_outputs]
  [CAN3_EVCCAplusPwrUpReq] -> bus_creator/1  "CAN3_EVCCAplusPwrUpReq"
  [CAN3_FDADC12VDet] -> bus_creator/2  "CAN3_FDADC12VDet"
  [CAN3_FDADC12VDetAvg] -> bus_creator/3  "CAN3_FDADC12VDetAvg"
  [CAN3_FDC_SYS_PmicBootPath] -> bus_creator/4  "CAN3_FDC_SYS_PmicBootPath"
  [CAN3_FDC_VCU_ActMaxSlideRate_Sta] -> bus_creator/5  "CAN3_FDC_VCU_ActMaxSlideRate_Sta"
  [CAN3_FDC_VCU_AllowMovThd_OTA_Sta] -> bus_creator/6  "CAN3_FDC_VCU_AllowMovThd_OTA_Sta"
  [CAN3_FDC_VCU_BOSEnable_Sta] -> bus_creator/7  "CAN3_FDC_VCU_BOSEnable_Sta"
  [CAN3_FDC_VCU_BrakeSigMatrix_Sta] -> bus_creator/8  "CAN3_FDC_VCU_BrakeSigMatrix_Sta"
  [CAN3_FDC_VCU_BrkPedalPosSta_Sta] -> bus_creator/9  "CAN3_FDC_VCU_BrkPedalPosSta_Sta"
  [CAN3_FDC_VCU_CANBrkSW2Sta_Sta] -> bus_creator/10  "CAN3_FDC_VCU_CANBrkSW2Sta_Sta"
  [CAN3_FDC_VCU_DTCCarousel_Sta] -> bus_creator/11  "CAN3_FDC_VCU_DTCCarousel_Sta"
  [CAN3_FDC_VCU_EAPS1Min_Sta] -> bus_creator/12  "CAN3_FDC_VCU_EAPS1Min_Sta"
  [CAN3_FDC_VCU_EAPS1Raw_Sta] -> bus_creator/13  "CAN3_FDC_VCU_EAPS1Raw_Sta"
  [CAN3_FDC_VCU_EAPS2Min_Sta] -> bus_creator/14  "CAN3_FDC_VCU_EAPS2Min_Sta"
  [CAN3_FDC_VCU_EAPS2Raw_Sta] -> bus_creator/15  "CAN3_FDC_VCU_EAPS2Raw_Sta"
  [CAN3_FDC_VCU_ForceP_Cmd] -> bus_creator/16  "CAN3_FDC_VCU_ForceP_Cmd"
  [CAN3_FDC_VCU_FrFirstOrderInpTs] -> bus_creator/17  "CAN3_FDC_VCU_FrFirstOrderInpTs"
  [CAN3_FDC_VCU_FrRateLimitDec_Sta] -> bus_creator/18  "CAN3_FDC_VCU_FrRateLimitDec_Sta"
  [CAN3_FDC_VCU_FrRateLimitInc_Sta] -> bus_creator/19  "CAN3_FDC_VCU_FrRateLimitInc_Sta"
  [CAN3_FDC_VCU_LVChrgFreqCnt_Sta] -> bus_creator/20  "CAN3_FDC_VCU_LVChrgFreqCnt_Sta"
  [CAN3_FDC_VCU_LVStaDropQukCnt_Sta] -> bus_creator/21  "CAN3_FDC_VCU_LVStaDropQukCnt_Sta"
  [CAN3_FDC_VCU_LowIdleAccPedal_Sta] -> bus_creator/22  "CAN3_FDC_VCU_LowIdleAccPedal_Sta"
  [CAN3_FDC_VCU_OTAPwrReqOFFChk_Sta] -> bus_creator/23  "CAN3_FDC_VCU_OTAPwrReqOFFChk_Sta"
  [CAN3_FDC_VCU_OTAPwrReqStdChk_Sta] -> bus_creator/24  "CAN3_FDC_VCU_OTAPwrReqStdChk_Sta"
  [CAN3_FDC_VCU_PwrReq_OTA_Sta] -> bus_creator/25  "CAN3_FDC_VCU_PwrReq_OTA_Sta"
  [CAN3_FDC_VCU_RWDRDCActive_Sta] -> bus_creator/26  "CAN3_FDC_VCU_RWDRDCActive_Sta"
  [CAN3_FDC_VCU_RegenTqLimitEn_Sta] -> bus_creator/27  "CAN3_FDC_VCU_RegenTqLimitEn_Sta"
  [CAN3_FDC_VCU_RrFirstOrderInpTs] -> bus_creator/28  "CAN3_FDC_VCU_RrFirstOrderInpTs"
  [CAN3_FDC_VCU_RrRateLimitDec_Sta] -> bus_creator/29  "CAN3_FDC_VCU_RrRateLimitDec_Sta"
  [CAN3_FDC_VCU_RrRateLimitInc_Sta] -> bus_creator/30  "CAN3_FDC_VCU_RrRateLimitInc_Sta"
  [CAN3_FDC_VCU_SlideRegenLimTq_Sta] -> bus_creator/31  "CAN3_FDC_VCU_SlideRegenLimTq_Sta"
  [CAN3_FDC_VCU_VehActSpd_Sta] -> bus_creator/32  "CAN3_FDC_VCU_VehActSpd_Sta"
  [CAN3_FDC_VCU_VehMalfunLevel_Sta] -> bus_creator/33  "CAN3_FDC_VCU_VehMalfunLevel_Sta"
  [CAN3_FDC_VMC_ActStESCYaw_Sta] -> bus_creator/34  "CAN3_FDC_VMC_ActStESCYaw_Sta"
  [CAN3_FDC_VMC_LongAcc_Sta] -> bus_creator/35  "CAN3_FDC_VMC_LongAcc_Sta"
  [CAN3_Fr_TqSource] -> bus_creator/36  "CAN3_Fr_TqSource"
  [CAN3_HVRlyOpFail] -> bus_creator/37  "CAN3_HVRlyOpFail"
  [CAN3_HVTHCMSysAvail] -> bus_creator/38  "CAN3_HVTHCMSysAvail"
  [CAN3_LVBattChrgtimeAct] -> bus_creator/39  "CAN3_LVBattChrgtimeAct"
  [CAN3_LVBattVoltSta] -> bus_creator/40  "CAN3_LVBattVoltSta"
  [CAN3_LVChrgHoldTAct] -> bus_creator/41  "CAN3_LVChrgHoldTAct"
  [CAN3_LVSilentChrgLv] -> bus_creator/42  "CAN3_LVSilentChrgLv"
  [CAN3_LVSilentChrgReq] -> bus_creator/43  "CAN3_LVSilentChrgReq"
  [CAN3_LVSilentChrgSta] -> bus_creator/44  "CAN3_LVSilentChrgSta"
  [CAN3_MCUActDisFail] -> bus_creator/45  "CAN3_MCUActDisFail"
  [CAN3_PMMAllowECUSleep] -> bus_creator/46  "CAN3_PMMAllowECUSleep"
  [CAN3_PmicBootReason] -> bus_creator/47  "CAN3_PmicBootReason"
  [CAN3_PowerDownFault] -> bus_creator/48  "CAN3_PowerDownFault"
  [CAN3_PowerDownState] -> bus_creator/49  "CAN3_PowerDownState"
  [CAN3_PowerUpFault] -> bus_creator/50  "CAN3_PowerUpFault"
  [CAN3_PowerUpState] -> bus_creator/51  "CAN3_PowerUpState"
  [CAN3_PwrDownReq] -> bus_creator/52  "CAN3_PwrDownReq"
  [CAN3_PwrStaConstraint] -> bus_creator/53  "CAN3_PwrStaConstraint"
  [CAN3_PwrStaONTOIVIPopReq] -> bus_creator/54  "CAN3_PwrStaONTOIVIPopReq"
  [CAN3_PwrStaONTOIVIPopT] -> bus_creator/55  "CAN3_PwrStaONTOIVIPopT"
  [CAN3_PwrStaSelect] -> bus_creator/56  "CAN3_PwrStaSelect"
  [CAN3_PwrStaTOSta] -> bus_creator/57  "CAN3_PwrStaTOSta"
  [CAN3_PwrUpReq] -> bus_creator/58  "CAN3_PwrUpReq"
  [CAN3_Rr_TqSource] -> bus_creator/59  "CAN3_Rr_TqSource"
  [CAN3_SchedChgTOSta] -> bus_creator/60  "CAN3_SchedChgTOSta"
  [CAN3_SilentChkAllowSleep] -> bus_creator/61  "CAN3_SilentChkAllowSleep"
  [CAN3_SysAllowReadySta] -> bus_creator/62  "CAN3_SysAllowReadySta"
  [CAN3_SysPwrSta] -> bus_creator/63  "CAN3_SysPwrSta"
  [CAN3_TCountSta] -> bus_creator/64  "CAN3_TCountSta"
  [CAN3_TimerAllowSleep] -> bus_creator/65  "CAN3_TimerAllowSleep"
  [CAN3_VCUBrkSWSta] -> bus_creator/66  "CAN3_VCUBrkSWSta"
  [CAN3_VCUFLDoorSta] -> bus_creator/67  "CAN3_VCUFLDoorSta"
  [CAN3_VCUFRDoorSta] -> bus_creator/68  "CAN3_VCUFRDoorSta"
  [CAN3_VCURLDoorSta] -> bus_creator/69  "CAN3_VCURLDoorSta"
  [CAN3_VCURRDoorSta] -> bus_creator/70  "CAN3_VCURRDoorSta"
  [CAN3_VehHVPwrAvail4THCM] -> bus_creator/71  "CAN3_VehHVPwrAvail4THCM"
  [CAN3_WisrBootReason] -> bus_creator/72  "CAN3_WisrBootReason"
  bus_creator/1 -> FD3_VCU0/1
  EVCCAplusPwrUpReq/1(CAN3_EVCCAplusPwrUpReq) -> [CAN3_EVCCAplusPwrUpReq]
  FDADC12VDet/1(CAN3_FDADC12VDet) -> [CAN3_FDADC12VDet]
  FDADC12VDetAvg/1(CAN3_FDADC12VDetAvg) -> [CAN3_FDADC12VDetAvg]
  FDCSYSPmicBootPath/1(CAN3_FDC_SYS_PmicBootPath) -> [CAN3_FDC_SYS_PmicBootPath]
  FDCVCUActMaxSlideRateSta/1(CAN3_FDC_VCU_ActMaxSlideRate_Sta) -> [CAN3_FDC_VCU_ActMaxSlideRate_Sta]
  FDCVCUAllowMovThdOTASta/1(CAN3_FDC_VCU_AllowMovThd_OTA_Sta) -> [CAN3_FDC_VCU_AllowMovThd_OTA_Sta]
  FDCVCUBOSEnableSta/1(CAN3_FDC_VCU_BOSEnable_Sta) -> [CAN3_FDC_VCU_BOSEnable_Sta]
  FDCVCUBrakeSigMatrixSta/1(CAN3_FDC_VCU_BrakeSigMatrix_Sta) -> [CAN3_FDC_VCU_BrakeSigMatrix_Sta]
  FDCVCUBrkPedalPosStaSta/1(CAN3_FDC_VCU_BrkPedalPosSta_Sta) -> [CAN3_FDC_VCU_BrkPedalPosSta_Sta]
  FDCVCUCANBrkSW2StaSta/1(CAN3_FDC_VCU_CANBrkSW2Sta_Sta) -> [CAN3_FDC_VCU_CANBrkSW2Sta_Sta]
  FDCVCUDTCCarouselSta/1(CAN3_FDC_VCU_DTCCarousel_Sta) -> [CAN3_FDC_VCU_DTCCarousel_Sta]
  FDCVCUEAPS1MinSta/1(CAN3_FDC_VCU_EAPS1Min_Sta) -> [CAN3_FDC_VCU_EAPS1Min_Sta]
  FDCVCUEAPS1RawSta/1(CAN3_FDC_VCU_EAPS1Raw_Sta) -> [CAN3_FDC_VCU_EAPS1Raw_Sta]
  FDCVCUEAPS2MinSta/1(CAN3_FDC_VCU_EAPS2Min_Sta) -> [CAN3_FDC_VCU_EAPS2Min_Sta]
  FDCVCUEAPS2RawSta/1(CAN3_FDC_VCU_EAPS2Raw_Sta) -> [CAN3_FDC_VCU_EAPS2Raw_Sta]
  FDCVCUForcePCmd/1(CAN3_FDC_VCU_ForceP_Cmd) -> [CAN3_FDC_VCU_ForceP_Cmd]
  FDCVCUFrFirstOrderInpTs/1(CAN3_FDC_VCU_FrFirstOrderInpTs) -> [CAN3_FDC_VCU_FrFirstOrderInpTs]
  FDCVCUFrRateLimitDecSta/1(CAN3_FDC_VCU_FrRateLimitDec_Sta) -> [CAN3_FDC_VCU_FrRateLimitDec_Sta]
  FDCVCUFrRateLimitIncSta/1(CAN3_FDC_VCU_FrRateLimitInc_Sta) -> [CAN3_FDC_VCU_FrRateLimitInc_Sta]
  FDCVCULVChrgFreqCntSta/1(CAN3_FDC_VCU_LVChrgFreqCnt_Sta) -> [CAN3_FDC_VCU_LVChrgFreqCnt_Sta]
  FDCVCULVStaDropQukCntSta/1(CAN3_FDC_VCU_LVStaDropQukCnt_Sta) -> [CAN3_FDC_VCU_LVStaDropQukCnt_Sta]
  FDCVCULowIdleAccPedalSta/1(CAN3_FDC_VCU_LowIdleAccPedal_Sta) -> [CAN3_FDC_VCU_LowIdleAccPedal_Sta]
  FDCVCUOTAPwrReqOFFChkSta/1(CAN3_FDC_VCU_OTAPwrReqOFFChk_Sta) -> [CAN3_FDC_VCU_OTAPwrReqOFFChk_Sta]
  FDCVCUOTAPwrReqStdChkSta/1(CAN3_FDC_VCU_OTAPwrReqStdChk_Sta) -> [CAN3_FDC_VCU_OTAPwrReqStdChk_Sta]
  FDCVCUPwrReqOTASta/1(CAN3_FDC_VCU_PwrReq_OTA_Sta) -> [CAN3_FDC_VCU_PwrReq_OTA_Sta]
  FDCVCURWDRDCActiveSta/1(CAN3_FDC_VCU_RWDRDCActive_Sta) -> [CAN3_FDC_VCU_RWDRDCActive_Sta]
  FDCVCURegenTqLimitEnSta/1(CAN3_FDC_VCU_RegenTqLimitEn_Sta) -> [CAN3_FDC_VCU_RegenTqLimitEn_Sta]
  FDCVCURrFirstOrderInpTs/1(CAN3_FDC_VCU_RrFirstOrderInpTs) -> [CAN3_FDC_VCU_RrFirstOrderInpTs]
  FDCVCURrRateLimitDecSta/1(CAN3_FDC_VCU_RrRateLimitDec_Sta) -> [CAN3_FDC_VCU_RrRateLimitDec_Sta]
  FDCVCURrRateLimitIncSta/1(CAN3_FDC_VCU_RrRateLimitInc_Sta) -> [CAN3_FDC_VCU_RrRateLimitInc_Sta]
  FDCVCUSlideRegenLimTqSta/1(CAN3_FDC_VCU_SlideRegenLimTq_Sta) -> [CAN3_FDC_VCU_SlideRegenLimTq_Sta]
  FDCVCUVehActSpdSta/1(CAN3_FDC_VCU_VehActSpd_Sta) -> [CAN3_FDC_VCU_VehActSpd_Sta]
  FDCVCUVehMalfunLevelSta/1(CAN3_FDC_VCU_VehMalfunLevel_Sta) -> [CAN3_FDC_VCU_VehMalfunLevel_Sta]
  FDCVMCActStESCYawSta/1(CAN3_FDC_VMC_ActStESCYaw_Sta) -> [CAN3_FDC_VMC_ActStESCYaw_Sta]
  FDCVMCLongAccSta/1(CAN3_FDC_VMC_LongAcc_Sta) -> [CAN3_FDC_VMC_LongAcc_Sta]
  FrTqSource/1(CAN3_Fr_TqSource) -> [CAN3_Fr_TqSource]
  HVRlyOpFail/1(CAN3_HVRlyOpFail) -> [CAN3_HVRlyOpFail]
  HVTHCMSysAvail/1(CAN3_HVTHCMSysAvail) -> [CAN3_HVTHCMSysAvail]
  LVBattChrgtimeAct/1(CAN3_LVBattChrgtimeAct) -> [CAN3_LVBattChrgtimeAct]
  LVBattVoltSta/1(CAN3_LVBattVoltSta) -> [CAN3_LVBattVoltSta]
  LVChrgHoldTAct/1(CAN3_LVChrgHoldTAct) -> [CAN3_LVChrgHoldTAct]
  LVSilentChrgLv/1(CAN3_LVSilentChrgLv) -> [CAN3_LVSilentChrgLv]
  LVSilentChrgReq/1(CAN3_LVSilentChrgReq) -> [CAN3_LVSilentChrgReq]
  LVSilentChrgSta/1(CAN3_LVSilentChrgSta) -> [CAN3_LVSilentChrgSta]
  MCUActDisFail/1(CAN3_MCUActDisFail) -> [CAN3_MCUActDisFail]
  PMMAllowECUSleep/1(CAN3_PMMAllowECUSleep) -> [CAN3_PMMAllowECUSleep]
  PmicBootReason/1(CAN3_PmicBootReason) -> [CAN3_PmicBootReason]
  PowerDownFault/1(CAN3_PowerDownFault) -> [CAN3_PowerDownFault]
  PowerDownState/1(CAN3_PowerDownState) -> [CAN3_PowerDownState]
  PowerUpFault/1(CAN3_PowerUpFault) -> [CAN3_PowerUpFault]
  PowerUpState/1(CAN3_PowerUpState) -> [CAN3_PowerUpState]
  PwrDownReq/1(CAN3_PwrDownReq) -> [CAN3_PwrDownReq]
  PwrStaConstraint/1(CAN3_PwrStaConstraint) -> [CAN3_PwrStaConstraint]
  PwrStaONTOIVIPopReq/1(CAN3_PwrStaONTOIVIPopReq) -> [CAN3_PwrStaONTOIVIPopReq]
  PwrStaONTOIVIPopT/1(CAN3_PwrStaONTOIVIPopT) -> [CAN3_PwrStaONTOIVIPopT]
  PwrStaSelect/1(CAN3_PwrStaSelect) -> [CAN3_PwrStaSelect]
  PwrStaTOSta/1(CAN3_PwrStaTOSta) -> [CAN3_PwrStaTOSta]
  PwrUpReq/1(CAN3_PwrUpReq) -> [CAN3_PwrUpReq]
  RrTqSource/1(CAN3_Rr_TqSource) -> [CAN3_Rr_TqSource]
  SchedChgTOSta/1(CAN3_SchedChgTOSta) -> [CAN3_SchedChgTOSta]
  SilentChkAllowSleep/1(CAN3_SilentChkAllowSleep) -> [CAN3_SilentChkAllowSleep]
  SysAllowReadySta/1(CAN3_SysAllowReadySta) -> [CAN3_SysAllowReadySta]
  SysPwrSta/1(CAN3_SysPwrSta) -> [CAN3_SysPwrSta]
  TCountSta/1(CAN3_TCountSta) -> [CAN3_TCountSta]
  TimerAllowSleep/1(CAN3_TimerAllowSleep) -> [CAN3_TimerAllowSleep]
  VCUBrkSWSta/1(CAN3_VCUBrkSWSta) -> [CAN3_VCUBrkSWSta]
  VCUFLDoorSta/1(CAN3_VCUFLDoorSta) -> [CAN3_VCUFLDoorSta]
  VCUFRDoorSta/1(CAN3_VCUFRDoorSta) -> [CAN3_VCUFRDoorSta]
  VCURLDoorSta/1(CAN3_VCURLDoorSta) -> [CAN3_VCURLDoorSta]
  VCURRDoorSta/1(CAN3_VCURRDoorSta) -> [CAN3_VCURRDoorSta]
  VehHVPwrAvail4THCM/1(CAN3_VehHVPwrAvail4THCM) -> [CAN3_VehHVPwrAvail4THCM]
  WisrBootReason/1(CAN3_WisrBootReason) -> [CAN3_WisrBootReason]
  bus_selector/1 -> EVCCAplusPwrUpReq/1(EVCCAplusPwrUpReq)  "<VOUTP_EvccAplusPwrUpReq_flg>"
  [BOUTP_outputs] -> bus_selector/1
  Ground/1 -> FDADC12VDet/1(FDADC12VDet)
  bus_selector1/1 -> FDADC12VDetAvg/1(FDADC12VDetAvg)  "<VOUTP_FDADC12VDetAvg_mV>"
  [BOUTP_outputs] -> bus_selector1/1
  bus_selector2/1 -> FDCSYSPmicBootPath/1(FDCSYSPmicBootPath)  "<VOUTP_PmicBootPath_raw32>"
  [BOUTP_outputs] -> bus_selector2/1
  bus_selector3/1 -> FDCVCUActMaxSlideRateSta/1(FDCVCUActMaxSlideRateSta)  "<VOUTP_MaxWhlSlideRate_pct>"
  [BOUTP_outputs] -> bus_selector3/1
  Ground1/1 -> FDCVCUAllowMovThdOTASta/1(FDCVCUAllowMovThdOTASta)
  bus_selector4/1 -> FDCVCUBOSEnableSta/1(FDCVCUBOSEnableSta)  "<VOUTP_BOSEnable_flg>"
  [BOUTP_outputs] -> bus_selector4/1
  Ground2/1 -> FDCVCUBrakeSigMatrixSta/1(FDCVCUBrakeSigMatrixSta)
  Ground3/1 -> FDCVCUBrkPedalPosStaSta/1(FDCVCUBrkPedalPosStaSta)
  Ground4/1 -> FDCVCUCANBrkSW2StaSta/1(FDCVCUCANBrkSW2StaSta)
  bus_selector5/1 -> FDCVCUDTCCarouselSta/1(FDCVCUDTCCarouselSta)  "<VOUTP_DTCDetect_enum>"
  [BOUTP_outputs] -> bus_selector5/1
  bus_selector6/1 -> FDCVCUEAPS1MinSta/1(FDCVCUEAPS1MinSta)  "<VOUTP_EAPS1MIN_pct>"
  [BOUTP_outputs] -> bus_selector6/1
  bus_selector7/1 -> FDCVCUEAPS2MinSta/1(FDCVCUEAPS2MinSta)  "<VOUTP_EAPS2MIN_pct>"
  [BOUTP_outputs] -> bus_selector7/1
  bus_selector8/1 -> FDCVCUForcePCmd/1(FDCVCUForcePCmd)  "<VOUTP_ForceP_flg>"
  [BOUTP_outputs] -> bus_selector8/1
  bus_selector9/1 -> FDCVCUFrFirstOrderInpTs/1(FDCVCUFrFirstOrderInpTs)  "<VOUTP_FrFirstOrderInpTs_c>"
  [BOUTP_outputs] -> bus_selector9/1
  bus_selector10/1 -> FDCVCUFrRateLimitDecSta/1(FDCVCUFrRateLimitDecSta)  "<VOUTP_FrRateLimitDec_Nm>"
  [BOUTP_outputs] -> bus_selector10/1
  bus_selector11/1 -> FDCVCUFrRateLimitIncSta/1(FDCVCUFrRateLimitIncSta)  "<VOUTP_FrRateLimitInc_Nm>"
  [BOUTP_outputs] -> bus_selector11/1
  Ground8/1 -> FDCVCULVStaDropQukCntSta/1(FDCVCULVStaDropQukCntSta)
  bus_selector12/1 -> FDCVCULowIdleAccPedalSta/1(FDCVCULowIdleAccPedalSta)  "<VOUTP_LowIdleAccPedal_flg>"
  [BOUTP_outputs] -> bus_selector12/1
  Ground9/1 -> FDCVCUOTAPwrReqOFFChkSta/1(FDCVCUOTAPwrReqOFFChkSta)
  Ground10/1 -> FDCVCUOTAPwrReqStdChkSta/1(FDCVCUOTAPwrReqStdChkSta)
  bus_selector13/1 -> FDCVCUPwrReqOTASta/1(FDCVCUPwrReqOTASta)  "<VOUTP_PwrReq_OTA_enum>"
  [BOUTP_outputs] -> bus_selector13/1
  bus_selector14/1 -> FDCVCURWDRDCActiveSta/1(FDCVCURWDRDCActiveSta)  "<VOUTP_RDCActive_enum>"
  [BOUTP_outputs] -> bus_selector14/1
  bus_selector15/1 -> FDCVCURegenTqLimitEnSta/1(FDCVCURegenTqLimitEnSta)  "<VOUTP_RegenTqLimitEn_flg>"
  [BOUTP_outputs] -> bus_selector15/1
  bus_selector16/1 -> FDCVCURrFirstOrderInpTs/1(FDCVCURrFirstOrderInpTs)  "<VOUTP_RrFirstOrderInpTs_c>"
  [BOUTP_outputs] -> bus_selector16/1
  bus_selector17/1 -> FDCVCURrRateLimitDecSta/1(FDCVCURrRateLimitDecSta)  "<VOUTP_RrRateLimitDec_Nm>"
  [BOUTP_outputs] -> bus_selector17/1
  bus_selector18/1 -> FDCVCURrRateLimitIncSta/1(FDCVCURrRateLimitIncSta)  "<VOUTP_RrRateLimitInc_Nm>"
  [BOUTP_outputs] -> bus_selector18/1
  bus_selector19/1 -> FDCVCUSlideRegenLimTqSta/1(FDCVCUSlideRegenLimTqSta)  "<VOUTP_SlideRegenLimTq_Nm>"
  [BOUTP_outputs] -> bus_selector19/1
  bus_selector20/1 -> FDCVCUVehActSpdSta/1(FDCVCUVehActSpdSta)  "<VOUTP_VehActSpd_kph>"
  [BOUTP_outputs] -> bus_selector20/1
  Ground11/1 -> FDCVCUVehMalfunLevelSta/1(FDCVCUVehMalfunLevelSta)
  bus_selector21/1 -> FDCVMCActStESCYawSta/1(FDCVMCActStESCYawSta)  "<VOUTP_ActStESCYaw_Dps>"
  [BOUTP_outputs] -> bus_selector21/1
  bus_selector22/1 -> FDCVMCLongAccSta/1(FDCVMCLongAccSta)  "<VOUTP_LongAcc_Gps>"
  [BOUTP_outputs] -> bus_selector22/1
  bus_selector23/1 -> FrTqSource/1(FrTqSource)  "<VOUTP_TqSourceFr_enum>"
  [BOUTP_outputs] -> bus_selector23/1
  bus_selector24/1 -> HVRlyOpFail/1(HVRlyOpFail)  "<VOUTP_HVRlyOpFail_flg>"
  [BOUTP_outputs] -> bus_selector24/1
  bus_selector25/1 -> HVTHCMSysAvail/1(HVTHCMSysAvail)  "<VOUTP_HVTHCMSysAvail_enum>"
  [BOUTP_outputs] -> bus_selector25/1
  bus_selector26/1 -> LVBattChrgtimeAct/1(LVBattChrgtimeAct)  "<VOUTP_LVBattChrgTimeCnt_s>"
  [BOUTP_outputs] -> bus_selector26/1
  bus_selector27/1 -> LVBattVoltSta/1(LVBattVoltSta)  "<VOUTP_LVBattVoltSta_enum>"
  [BOUTP_outputs] -> bus_selector27/1
  bus_selector28/1 -> LVChrgHoldTAct/1(LVChrgHoldTAct)  "<VOUTP_LVChrgHoldTtimer_s>"
  [BOUTP_outputs] -> bus_selector28/1
  bus_selector29/1 -> LVSilentChrgLv/1(LVSilentChrgLv)  "<VOUTP_LVSilentChrgLv_enum>"
  [BOUTP_outputs] -> bus_selector29/1
  bus_selector30/1 -> LVSilentChrgReq/1(LVSilentChrgReq)  "<VOUTP_LVSilentChrgReq_flg>"
  [BOUTP_outputs] -> bus_selector30/1
  bus_selector31/1 -> LVSilentChrgSta/1(LVSilentChrgSta)  "<VOUTP_LVSilentChrgSta_enum>"
  [BOUTP_outputs] -> bus_selector31/1
  bus_selector32/1 -> MCUActDisFail/1(MCUActDisFail)  "<VOUTP_MCUActDisFail_flg>"
  [BOUTP_outputs] -> bus_selector32/1
  bus_selector33/1 -> PMMAllowECUSleep/1(PMMAllowECUSleep)  "<VOUTP_PMMAllowECUSleep_flg>"
  [BOUTP_outputs] -> bus_selector33/1
  bus_selector34/1 -> PmicBootReason/1(PmicBootReason)  "<VOUTP_PmicBootReason_enum>"
  [BOUTP_outputs] -> bus_selector34/1
  bus_selector35/1 -> PowerDownFault/1(PowerDownFault)  "<VOUTP_PowerDownFault_enum>"
  [BOUTP_outputs] -> bus_selector35/1
  bus_selector36/1 -> PowerDownState/1(PowerDownState)  "<VOUTP_PowerDownState_enum>"
  [BOUTP_outputs] -> bus_selector36/1
  bus_selector37/1 -> PowerUpFault/1(PowerUpFault)  "<VOUTP_PowerUpFault_enum>"
  [BOUTP_outputs] -> bus_selector37/1
  bus_selector38/1 -> PowerUpState/1(PowerUpState)  "<VOUTP_PowerUpState_enum>"
  [BOUTP_outputs] -> bus_selector38/1
  bus_selector39/1 -> PwrDownReq/1(PwrDownReq)  "<VOUTP_PwrDownReq_enum>"
  [BOUTP_outputs] -> bus_selector39/1
  bus_selector40/1 -> PwrStaConstraint/1(PwrStaConstraint)  "<VOUTP_PwrStaConstraint_enum>"
  [BOUTP_outputs] -> bus_selector40/1
  bus_selector41/1 -> PwrStaONTOIVIPopReq/1(PwrStaONTOIVIPopReq)  "<VOUTP_PwrStaONTOPopReq_flg>"
  [BOUTP_outputs] -> bus_selector41/1
  bus_selector42/1 -> PwrStaONTOIVIPopT/1(PwrStaONTOIVIPopT)  "<VOUTP_IVIPwrStaONTOPopT_s>"
  [BOUTP_outputs] -> bus_selector42/1
  bus_selector43/1 -> PwrStaSelect/1(PwrStaSelect)  "<VOUTP_PwrStaSelect_enum>"
  [BOUTP_outputs] -> bus_selector43/1
  bus_selector44/1 -> PwrStaTOSta/1(PwrStaTOSta)  "<VOUTP_PwrStaTOSta_enum>"
  [BOUTP_outputs] -> bus_selector44/1
  bus_selector45/1 -> PwrUpReq/1(PwrUpReq)  "<VOUTP_PwrUpReq_enum>"
  [BOUTP_outputs] -> bus_selector45/1
  bus_selector46/1 -> RrTqSource/1(RrTqSource)  "<VOUTP_TqSourceRr_enum>"
  [BOUTP_outputs] -> bus_selector46/1
  Ground12/1 -> SchedChgTOSta/1(SchedChgTOSta)
  bus_selector47/1 -> SilentChkAllowSleep/1(SilentChkAllowSleep)  "<VOUTP_SilentChkAllowSleep_flg>"
  [BOUTP_outputs] -> bus_selector47/1
  bus_selector48/1 -> SysAllowReadySta/1(SysAllowReadySta)  "<VOUTP_SysAllowReadySta_flg>"
  [BOUTP_outputs] -> bus_selector48/1
  bus_selector49/1 -> SysPwrSta/1(SysPwrSta)  "<VOUTP_SysPowerMode_enum>"
  [BOUTP_outputs] -> bus_selector49/1
  bus_selector50/1 -> TCountSta/1(TCountSta)  "<VOUTP_TCountSta_enum>"
  [BOUTP_outputs] -> bus_selector50/1
  bus_selector51/1 -> TimerAllowSleep/1(TimerAllowSleep)  "<VOUTP_TimerAllowSleep_flg>"
  [BOUTP_outputs] -> bus_selector51/1
  bus_selector52/1 -> VCUBrkSWSta/1(VCUBrkSWSta)  "<VOUTP_VCUBrkSWSta_enum>"
  [BOUTP_outputs] -> bus_selector52/1
  bus_selector53/1 -> VCUFLDoorSta/1(VCUFLDoorSta)  "<VOUTP_VCUFLDoorSta_flg>"
  [BOUTP_outputs] -> bus_selector53/1
  bus_selector54/1 -> VCUFRDoorSta/1(VCUFRDoorSta)  "<VOUTP_VCUFRDoorSta_flg>"
  [BOUTP_outputs] -> bus_selector54/1
  bus_selector55/1 -> VCURLDoorSta/1(VCURLDoorSta)  "<VOUTP_VCURLDoorSta_flg>"
  [BOUTP_outputs] -> bus_selector55/1
  bus_selector56/1 -> VCURRDoorSta/1(VCURRDoorSta)  "<VOUTP_VCURRDoorSta_flg>"
  [BOUTP_outputs] -> bus_selector56/1
  bus_selector57/1 -> VehHVPwrAvail4THCM/1(VehHVPwrAvail4THCM)  "<VOUTP_VehHVPwrAvail4THCM_W>"
  [BOUTP_outputs] -> bus_selector57/1
  bus_selector58/1 -> WisrBootReason/1(WisrBootReason)  "<VOUTP_WisrBootReason_raw32>"
  [BOUTP_outputs] -> bus_selector58/1
  [BOUTP_outputs] -> bus_selector59/1
  Data Type Conversion2/1 -> Subsystem/4(VOUTP_OTAPwrReqStdChkSta_enum)
  bus_selector59/2 -> Data Type Conversion1/1  "<VOUTP_OTAPwrReqOFFChkSta_enum>"
  Data Type Conversion/1 -> Subsystem/2(VOUTP_CurrentNmState_enum)
  s8_AcoreReadyToSleep/1 -> Subsystem/1(s8_AcoreReadyToSleep)
  bus_selector59/3 -> Data Type Conversion2/1  "<VOUTP_OTAPwrReqStdChkSta_enum>"
  Data Type Conversion1/1 -> Subsystem/3(VOUTP_OTAPwrReqOFFChkSta_enum)
  bus_selector59/1 -> Data Type Conversion/1  "<VOUTP_CurrentNmState_enum>"
  Subsystem/1(VehHVPwrAvail4THCM) -> FDCVCULVChrgFreqCntSta/1(FDCVCULVChrgFreqCntSta)
  [BOUTP_outputs] -> bus_selector60/1
  bus_selector60/1 -> FDCVCUEAPS2RawSta/1(FDCVCUEAPS2RawSta)  "<VOUTP_EAPS2RAW_pct>"
  [BOUTP_outputs] -> bus_selector61/1
  bus_selector61/1 -> FDCVCUEAPS1RawSta/1(FDCVCUEAPS1RawSta)  "<VOUTP_EAPS1RAW_pct>"
